simulink model "EV_50hp_DC_Motor"  (R2023a)
settings: Solver=ode45  StartTime=0.0  StopTime=200  RelTol=1e-3  EnableMultiTasking=on
libraries: spsDCMachineLib x1, simulink x1, spsControlledVoltageSourceLib x1, spsDCVoltageSourceLib x1, sps_lib x1
settings Model: Creator=INTEL  LastModifiedBy=kapilsharma
settings SolverCC: AlgebraicLoopSolver=LineSearch
settings DataIOCC: LimitDataPoints=on  SaveFormat=Array  ReturnWorkspaceOutputs=off
settings OptimizationCC: LifeSpan=inf
settings DebuggingCC: SolverPrmCheckMsg=warning  UnconnectedInputMsg=warning  UnconnectedOutputMsg=warning  UnconnectedLineMsg=warning  SFUnexpectedBacktrackingDiag=warning  SFNoUnconditionalDefaultTransitionDiag=warning  SFExecutionAtInitializationDiag=none  ArithmeticOperatorsInVariantConditions=warning
settings HardwareCC: ProdBitPerPointer=32  ProdBitPerSizeT=32  ProdBitPerPtrDiffT=32  ProdLargestAtomicFloat=None  ProdIntDivRoundTo=Undefined  ProdEndianess=Unspecified  ProdWordSize=32  ProdHWDeviceType=32-bit Generic
settings ModelReferenceCC: PropagateSignalLabelsOutOfModel=off
settings SFSimCC: SimUseLocalCustomCode=off  CustomCodeUndefinedFunction=UseInterfaceOnly
settings RTWCC: RTWUseLocalCustomCode=off
settings CodeAppCC: StateflowObjectComments=on
settings GRTTargetCC: TargetLangStandard=C89/C90 (ANSI)
settings ConfigComp: CovMetricSettings=dw  CovSaveCumulativeToWorkspaceVar=on  CovSaveSingleToWorkspaceVar=on  CovExternalEMLEnable=off  CovSFcnEnable=off
settings SimscapeCC: SimscapeNormalizeSystem=off

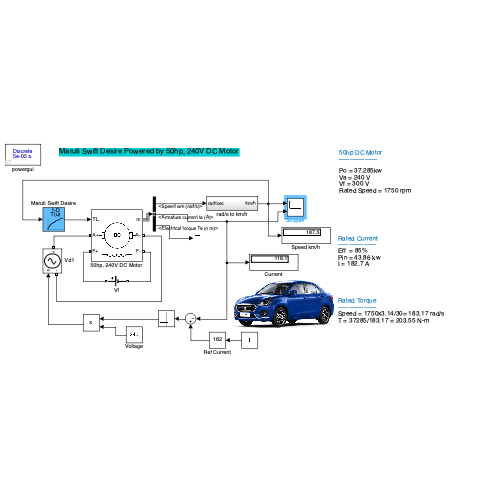
[thumbnail: Simulink's stored preview of the top-level diagram]
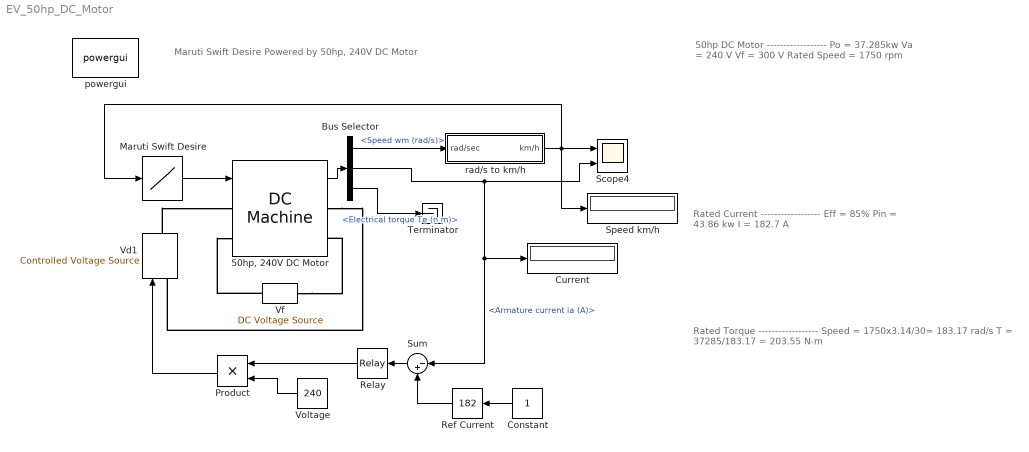
== system EV_50hp_DC_Motor ==
  note: Maruti Swift Desire Powered by 50hp, 240V DC Motor
  note: 50hp DC Motor
      | ------------------
      |
      | Po = 37.285kw
      | Va = 240 V
      | Vf = 300 V
      | Rated Speed = 1750 rpm
  note: Rated Current
      | ------------------
      | Eff = 85%
      | Pin = 43.86 kw
      | I = 182.7 A
  note: Rated Torque
      | ------------------
      | Speed = 1750x3.14/30= 183.17 rad/s
      | T = 37285/183.17 = 203.55 N-m
  "50hp, 240V DC Motor" : spsDCMachineLib/DC Machine  PresetModel=No  MechanicalLoad=Torque TL  FieldType=Wound  ShowDetailedParameters=on  MeasurementBus=off  RLa="[ 0.13  0.001558]"  RLf=[ 84.91 13.39]  Laf=0.3406  MachineConstant=Torque constant (N.m/A)  Ke=1.8  Kt=1.8  J=1335*0.279*0.279  Bm=0.007032  Tf=5.282  w0=1  Ifinit=3.53315274997056  TsPowergui=0  TsBlock=-1
  Bus Selector : BusSelector  OutputSignals=Speed wm (rad/s),Armature current ia (A),Electrical torque Te (n m)
  Constant : Constant
  Current : Display
  Maruti Swift Desire : Lookup_n-D  NumberOfTableDimensions=1  BreakpointsForDimension1=[0, 5, 10, 15, 20, 25, 30, 35, 40, 45, 50, 55, 60, 65, 70, 75, 80, 85, 90, 95, 100, 110, 120, 130, 140, 150, 160, 170, 180, 190, 200]  Table=[0, 16.65, 27.53, 35.7, 42.34, 48.02, 53.4, 57.58, 61.76, 65.65, 69.3, 72.76, 76.05, 79.19, 82.21, 85.12, 87.93, 90.65, 93.29, 95.86, 98.35, 103.2, 107.8, 112.2, 116.4, 120.5, 124.4, 128.3, 132, 135.6, 139.1]  InternalRulePriority=Speed  RndMeth=Simplest
  Product : Product
  Ref Current : simulink/Math Operations/Slider Gain  gain=182  low=0  high=187
  Relay : Relay  OnSwitchValue=2  OffSwitchValue=-2
  Scope4 : Scope  NumInputPorts=2
  Speed km/h : Display
  Sum : Sum  Inputs=|-+
  Terminator : Terminator
  Vd1 : spsControlledVoltageSourceLib/Controlled Voltage Source  Initialize=on  Source_Type=DC  Amplitude=0  Phase=0  Frequency=0  Measurements=None
  Vf : spsDCVoltageSourceLib/DC Voltage Source  Amplitude=300  Measurements=None
  Voltage : Constant  Value=240
  powergui : sps_lib/powergui  Priority=1  SimulationMode=Discrete  SampleTime=50e-6  frequency=60  Iterations=50  frequencyindice=0  Pbase=100e6  ErrMax=1e-4  UnitsV=kV  UnitsW=MW  buscounter=0  FunctionMessages=off  echomessages=off  EnableUseOfTLC=off  CurrentSourceSwitches=off  DisableSnubberDevices=off  DisableRonSwitches=off  DisableVfSwitches=off  DisplayEquations=off  AutomaticDiscreteSolvers=off  SolverType=Tustin/Backward Euler (TBE)  Interpol=off  ExternalGateDelay=off  methode=off  Ts=100  x0status=blocks  SPID=off  SwTol=0  HookPort=off  NonlinearTolerance=1e-4  nMaxIteration=100  ContinueOnMaxIteration=off  RestoreLinks=warning  ResistiveCurrentMeasurement=off  Frange=[0:2:500]  Ylog=off  Xlog=on  ShowGrid=off  save=off  variable=ZData  structure=0  ZoomFFT=off  StartTime=0.0  cycles=1  DisplayStyle=1  fundamental=60  FreqAxis=off  MaxFrequency=1000  frequencyindicesteady=1  RmsSteady=1  display=off
  rad/s to km/h : Subsystem
  wires:
  Maruti Swift Desire/1 -> "50hp, 240V DC Motor"/1
  "50hp, 240V DC Motor"/1 -> Bus Selector/1
  rad/s to km/h/1(km/h) -> Speed km/h/1, Scope4/1, Maruti Swift Desire/1
  Bus Selector/1 -> rad/s to km/h/1(rad/sec)  "<Speed wm (rad/s)>"
  Bus Selector/3 -> Terminator/1  "<Electrical torque Te (n m)>"
  Bus Selector/2 -> Sum/1, Current/1, Scope4/2  "<Armature current ia (A)>"
  Constant/1 -> Ref Current/1
  Sum/1 -> Relay/1
  Relay/1 -> Product/1
  Voltage/1 -> Product/2
  Product/1 -> Vd1/1
  Ref Current/1 -> Sum/2
  connections:
  Vf/RConn1 -- "50hp, 240V DC Motor"/LConn2
  Vf/LConn1 -- "50hp, 240V DC Motor"/RConn2
  Vd1/RConn1 -- "50hp, 240V DC Motor"/LConn1
  "50hp, 240V DC Motor"/RConn1 -- Vd1/LConn1

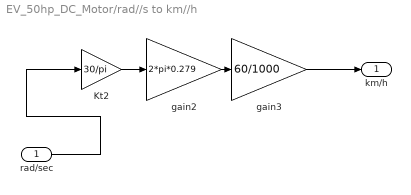
== system EV_50hp_DC_Motor/rad//s to km//h ==
  rad/sec : Inport
  Kt2 : Gain  Gain=30/pi
  gain2 : Gain  Gain=2*pi*0.279
  gain3 : Gain  Gain=60/1000
  km/h : Outport
  wires:
  Kt2/1 -> gain2/1
  gain2/1 -> gain3/1
  gain3/1 -> km/h/1
  rad/sec/1 -> Kt2/1
